simulink model "Model_Boost"  (R2024a)
settings: Solver=FixedStepDiscrete  StartTime=0.0  StopTime=5  FixedStep=1e-6  RelTol=1e-3  EnableMultiTasking=on
InitFcn:
  | Vin=20;
  | D=0.5;
  | fsw=10e3;
  | L=3.5e-3;
  | C=572e-6;
  | R=200;
  | Ts=1e-6;
libraries: spsCurrentMeasurementLib x4, spsVoltageMeasurementLib x3, spsParallelRLCBranchLib x2, spsSeriesRLCBranchLib x2, spsDCVoltageSourceLib x1, spsDiodeLib x1, spsMeanLib x1, spsMosfetLib x1, spsPWMGeneratorDCDCLib x1, simulink x1, spspowerguiLib x1
settings Model: Creator=NHN  LastModifiedBy=saqib
settings SolverCC: AlgebraicLoopSolver=TrustRegion
settings DataIOCC: LimitDataPoints=on  SaveFormat=Array  ReturnWorkspaceOutputs=off
settings OptimizationCC: LifeSpan=inf
settings DebuggingCC: UnderspecifiedInitializationDetection=Classic  MergeDetectMultiDrivingBlocksExec=none  SolverPrmCheckMsg=warning  UnconnectedInputMsg=warning  UnconnectedOutputMsg=warning  UnconnectedLineMsg=warning  StateNameClashWarn=warning  SFUnexpectedBacktrackingDiag=warning  SFNoUnconditionalDefaultTransitionDiag=warning  SFExecutionAtInitializationDiag=none  ArithmeticOperatorsInVariantConditions=warning
settings HardwareCC: ProdBitPerPointer=32  ProdBitPerSizeT=32  ProdBitPerPtrDiffT=32  ProdLargestAtomicFloat=None  ProdIntDivRoundTo=Undefined  ProdEndianess=Unspecified  ProdWordSize=32  ProdHWDeviceType=32-bit Generic
settings ModelReferenceCC: EnableRefExpFcnMdlSchedulingChecks=on  PropagateSignalLabelsOutOfModel=off
settings SFSimCC: SimUseLocalCustomCode=off  CustomCodeUndefinedFunction=UseInterfaceOnly
settings RTWCC: RTWUseLocalCustomCode=off  GPUComputeCapability=3.5
settings CodeAppCC: StateflowObjectComments=on
settings GRTTargetCC: TargetLangStandard=C89/C90 (ANSI)
settings ConfigComp: CovMetricSettings=dw  CovSaveCumulativeToWorkspaceVar=on  CovSaveSingleToWorkspaceVar=on  CovExternalEMLEnable=off
settings SimscapeCC: SimscapeNormalizeSystem=off

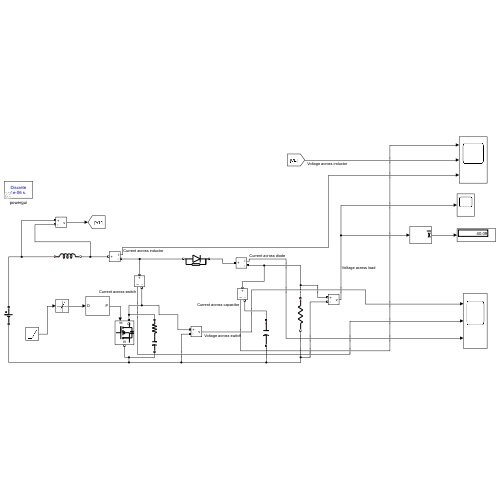
[thumbnail: Simulink's stored preview of the top-level diagram]
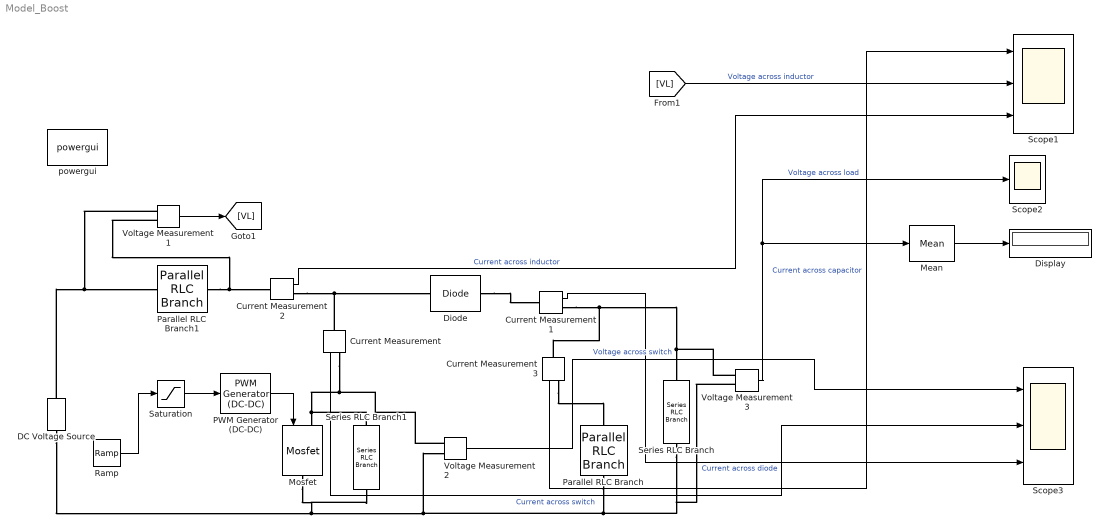
== system Model_Boost ==
  Current Measurement{,1..3} (4 alike) : spsCurrentMeasurementLib/Current Measurement  PhasorSimulation=off  OutputType=Complex  PSBequivalent=0
  DC Voltage Source : spsDCVoltageSourceLib/DC Voltage Source  Amplitude=20  Measurements=None
  Diode : spsDiodeLib/Diode  Ron=0.001  Lon=0  Vf=0.8  IC=0  UseSnubber=off  Rs=500  Cs=250e-9  Measurements=off
  Display : Display
  Mean : spsMeanLib/Mean  Freq=10000  Vinit=0  Ts=1e-6
  Mosfet : spsMosfetLib/Mosfet  Ron=0.1  Lon=0  Rd=0.01  Vfd=0  IC=0  Rs=1e5  Cs=inf  Measurements=off
  PWM Generator (DC-DC) : spsPWMGeneratorDCDCLib/PWM Generator (DC-DC)  Fsw=10e3  Ts=1e-6
  Parallel RLC Branch : spsParallelRLCBranchLib/Parallel RLC Branch  LConnTagsString=a  RConnTagsString=__new0  BranchType=C  Resistance=1  Inductance=1e-3  SetiL0=off  InitialCurrent=0  Capacitance=572e-6  Setx0=on  InitialVoltage=20  Measurements=None
  Parallel RLC Branch1 : spsParallelRLCBranchLib/Parallel RLC Branch  LConnTagsString=a  RConnTagsString=__new0  BranchType=L  Resistance=1  Inductance=3.5e-3  SetiL0=off  InitialCurrent=0  Capacitance=1e-6  Setx0=off  InitialVoltage=0  Measurements=None
  Ramp : simulink/Sources/Ramp  slope=5  start=0  InitialOutput=0
  Saturation : Saturate  LowerLimit=0
  Scope1 : Scope  NumInputPorts=3
  Scope2 : Scope
  Scope3 : Scope  NumInputPorts=3
  Series RLC Branch : spsSeriesRLCBranchLib/Series RLC Branch  LConnTagsString=__new0  RConnTagsString=__new0  BranchType=R  Resistance=200  Inductance=1e-3  SetiL0=off  InitialCurrent=0  Capacitance=1e-6  Setx0=off  InitialVoltage=0  Measurements=None
  Series RLC Branch1 : spsSeriesRLCBranchLib/Series RLC Branch  LConnTagsString=__new0  RConnTagsString=__new0  BranchType=RC  Resistance=1  Inductance=1e-3  SetiL0=off  InitialCurrent=0  Capacitance=1e-9  Setx0=off  InitialVoltage=0  Measurements=None
  Voltage Measurement1 : spsVoltageMeasurementLib/Voltage Measurement  PhasorSimulation=off  OutputType=Complex  PSBequivalent=0
  Voltage Measurement2 : spsVoltageMeasurementLib/Voltage Measurement  PhasorSimulation=off  OutputType=Complex  PSBequivalent=0
  Voltage Measurement3 : spsVoltageMeasurementLib/Voltage Measurement  PhasorSimulation=off  OutputType=Complex  PSBequivalent=0
  powergui : spspowerguiLib/powergui  Priority=1  SimulationMode=Discrete  SampleTime=1e-6  frequency=60  Iterations=50  frequencyindice=0  Pbase=100e6  ErrMax=1e-4  UnitsV=kV  UnitsW=MW  buscounter=0  FunctionMessages=off  echomessages=off  EnableUseOfTLC=off  CurrentSourceSwitches=off  DisableSnubberDevices=off  DisableRonSwitches=off  DisableVfSwitches=off  DisplayEquations=off  AutomaticDiscreteSolvers=off  SolverType=Tustin  Interpol=off  ExternalGateDelay=off  methode=off  Ts=0  x0status=blocks  SPID=off  SwTol=0  HookPort=off  NonlinearTolerance=1e-4  nMaxIteration=100  ContinueOnMaxIteration=off  RestoreLinks=warning  ResistiveCurrentMeasurement=off  Frange=[0:2:500]  Ylog=off  Xlog=on  ShowGrid=off  save=off  variable=ZData  structure=0  ZoomFFT=off  StartTime=0.0  cycles=1  DisplayStyle=1  fundamental=60  FreqAxis=off  MaxFrequency=1000  frequencyindicesteady=1  RmsSteady=1  display=off
  wires:
  PWM Generator (DC-DC)/1 -> Mosfet/1
  Current Measurement3/1 -> Scope1/1  "Current across capacitor"
  Voltage Measurement1/1 -> [VL]
  [VL] -> Scope1/2  "Voltage across inductor"
  Current Measurement2/1 -> Scope1/3  "Current across inductor"
  Voltage Measurement3/1 -> Scope2/1, Mean/1  "Voltage across load"
  Voltage Measurement2/1 -> Scope3/1  "Voltage across switch"
  Current Measurement/1 -> Scope3/2  "Current across switch"
  Current Measurement1/1 -> Scope3/3  "Current across diode"
  Mean/1 -> Display/1
  Ramp/1 -> Saturation/1
  Saturation/1 -> PWM Generator (DC-DC)/1
  connections:
  DC Voltage Source/RConn1 -- Voltage Measurement1/LConn1 -- Parallel RLC Branch1/LConn1
  Parallel RLC Branch1/RConn1 -- Voltage Measurement1/LConn2 -- Current Measurement2/LConn1
  Current Measurement2/RConn1 -- Diode/LConn1 -- Current Measurement/LConn1
  Current Measurement/RConn1 -- Voltage Measurement2/LConn1 -- Series RLC Branch1/LConn1 -- Mosfet/LConn1
  DC Voltage Source/LConn1 -- Series RLC Branch1/RConn1 -- Mosfet/RConn1 -- Voltage Measurement3/LConn2 -- Series RLC Branch/RConn1 -- Parallel RLC Branch/RConn1 -- Voltage Measurement2/LConn2
  Diode/RConn1 -- Current Measurement1/LConn1
  Current Measurement1/RConn1 -- Current Measurement3/LConn1 -- Voltage Measurement3/LConn1 -- Series RLC Branch/LConn1
  Current Measurement3/RConn1 -- Parallel RLC Branch/LConn1
